simulink library "csu_elc_execute_lc_commands_lib"  (R2014b)
settings: Solver=ode45  StartTime=0.0  StopTime=10.0  RelTol=1e-3
undefined symbols (not defined in the file or in its folder): lc_msgid
libraries: simulink x2, util_info_lib x1
settings Model: Creator=escrane  LastModifiedBy=mstewart

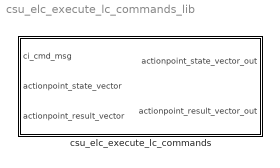
== system csu_elc_execute_lc_commands_lib ==
  csu_elc_execute_lc_commands : Subsystem

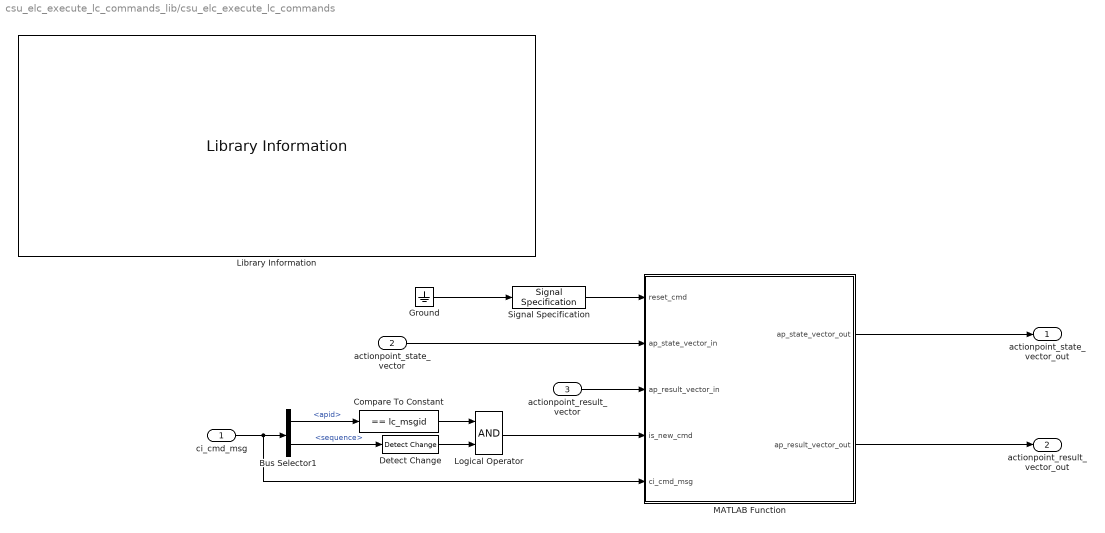
== system csu_elc_execute_lc_commands_lib/csu_elc_execute_lc_commands ==
  ci_cmd_msg : Inport
  actionpoint_state_vector : Inport  Port=2
  actionpoint_result_vector : Inport  Port=3
  Bus Selector1 : BusSelector  OutputSignals=apid,sequence
  Compare To Constant : simulink/Logic and Bit Operations/Compare To Constant  relop===  const=lc_msgid  OutDataTypeStr=boolean
  Detect Change : simulink/Logic and Bit Operations/Detect Change  vinit=0  InputProcessing=Inherited  OutDataTypeStr=boolean
  Ground : Ground
  Library Information : util_info_lib/Library Information  owner='escrane'
  Logical Operator : Logic  AllPortsSameDT=off  OutDataTypeStr=boolean
  MATLAB Function : MATLAB Function  TreatAsAtomicUnit=on
  Signal Specification : SignalSpecification  OutDataTypeStr=uint8
  actionpoint_state_vector_out : Outport
  actionpoint_result_vector_out : Outport  Port=2
  wires:
  Ground/1 -> Signal Specification/1
  ci_cmd_msg/1 -> MATLAB Function/5(ci_cmd_msg), Bus Selector1/1
  Bus Selector1/1 -> Compare To Constant/1  "<apid>"
  Bus Selector1/2 -> Detect Change/1  "<sequence>"
  Compare To Constant/1 -> Logical Operator/1
  Detect Change/1 -> Logical Operator/2
  Logical Operator/1 -> MATLAB Function/4(is_new_cmd)
  actionpoint_state_vector/1 -> MATLAB Function/2(ap_state_vector_in)
  MATLAB Function/1(ap_state_vector_out) -> actionpoint_state_vector_out/1
  actionpoint_result_vector/1 -> MATLAB Function/3(ap_result_vector_in)
  MATLAB Function/2(ap_result_vector_out) -> actionpoint_result_vector_out/1
  Signal Specification/1 -> MATLAB Function/1(reset_cmd)

== matlab function csu_elc_execute_lc_commands_lib/csu_elc_execute_lc_commands/MATLAB Function ==
  data: reset_cmd input; ap_state_vector_out output uint8; ap_state_vector_in input; ap_result_vector_in input; is_new_cmd input; ci_cmd_msg input; ap_result_vector_out output boolean
function [ap_state_vector_out,ap_result_vector_out]  = lc_command_ingest(reset_cmd, ap_state_vector_in,ap_result_vector_in, is_new_cmd, ci_cmd_msg)
%#codegen

ap_state_vector_out  = ap_state_vector_in;
ap_result_vector_out = ap_result_vector_in;



if is_new_cmd

    %%% Handle change state commands
    if (ci_cmd_msg.command_id == 4)
        
        actionpoint_id = typecast(ci_cmd_msg.params(1),'uint8');   
        new_state = typecast(ci_cmd_msg.params(2),'uint8');   
        
        ap_state_vector_out( actionpoint_id ) = new_state; 
        
    end
 
end
